simulink model "flightControlSystem"  (R2021a)
settings: Solver=ode3  StartTime=0  StopTime=TFinal  FixedStep=Ts  RelTol=1e-3  EnableMultiTasking=on
undefined symbols (not defined in the file): codertarget, Estimator, Ts
libraries: simulink x6
settings Model: ExtModeTrigDuration=80  Creator=The MathWorks, Inc.  LastModifiedBy=s2130866
settings SolverCC: AlgebraicLoopSolver=TrustRegion
settings DataIOCC: LimitDataPoints=on  SaveFormat=StructureWithTime  ReturnWorkspaceOutputs=off
settings OptimizationCC: BlockReduction=off  EnhancedBackFolding=on  PassReuseOutputArgsAs=Individual arguments  ZeroExternalMemoryAtStartup=off  ZeroInternalMemoryAtStartup=off  MaxStackSize=64  OptimizeBlockOrder=speed  DifferentSizesBufferReuse=on  OptimizationCustomize=off  EfficientTunableParamExpr=on
settings DebuggingCC: AlgebraicLoopMsg=none  IntegerOverflowMsg=none  ParameterPrecisionLossMsg=none  ParameterTunabilityLossMsg=error  UnconnectedInputMsg=none  UnconnectedOutputMsg=none  UnconnectedLineMsg=none  BusObjectLabelMismatch=error  SFUnexpectedBacktrackingDiag=warning  SFNoUnconditionalDefaultTransitionDiag=warning  SFExecutionAtInitializationDiag=none  SFMachineParentedDataDiag=warning  IntegerSaturationMsg=none  ArithmeticOperatorsInVariantConditions=warning
settings HardwareCC: ProdBitPerPointer=32  ProdBitPerSizeT=32  ProdBitPerPtrDiffT=32  ProdLargestAtomicInteger=Long  ProdWordSize=32  ProdHWDeviceType=ARM Compatible->ARM 9
settings ModelReferenceCC: ModelReferenceNumInstancesAllowed=Single  PropagateSignalLabelsOutOfModel=off
settings SFSimCC: SimUseLocalCustomCode=off  MATLABDynamicMemAlloc=off  CustomCodeUndefinedFunction=UseInterfaceOnly
settings RTWCC: SystemTargetFile=ert.tlc  HardwareBoard=PARROT Mambo  TemplateMakefile=ert_default_tmf  GenerateReport=on  RTWUseLocalCustomCode=off  Toolchain=Sourcery G++ Lite GNU Toolchain for Drones  LaunchReport=on
settings CodeAppCC: ForceParamTrailComments=on  IgnoreCustomStorageClasses=off  MaxIdLength=63  OperatorAnnotations=on  SimulinkDataObjDesc=on  SFDataObjDesc=on  InsertBlockDesc=on
settings ERTTargetCC: MatFileLogging=on
settings ConfigComp: CovMetricSettings=dw  CovSaveCumulativeToWorkspaceVar=on  CovSaveSingleToWorkspaceVar=on  CovExternalEMLEnable=off  CovSFcnEnable=off

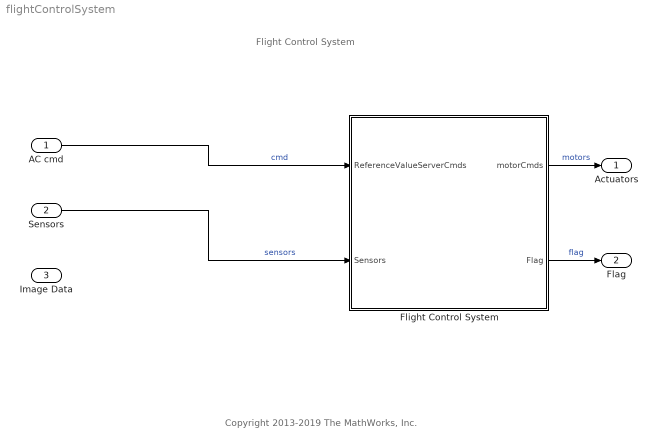
== system flightControlSystem ==
  note: Copyright 2013-2019 The MathWorks, Inc.
  note: Flight Control System
  AC cmd : Inport  OutDataTypeStr=Bus: CommandBus  BusOutputAsStruct=on
  Sensors : Inport  Port=2  OutDataTypeStr=Bus: SensorsBus  BusOutputAsStruct=on
  Image Data : Inport  Tag=IP_IN  InitFcn=codertarget.parrot.internal.inportCallback(gcb);  Port=3  OutDataTypeStr=uint8  PortDimensions=[4 9600]  BusOutputAsStruct=on
  Flight Control System : Subsystem  TreatAsAtomicUnit=on  SystemSampleTime=Ts
  Actuators : Outport  OutDataTypeStr=single  PortDimensions=4  VectorParamsAs1DForOutWhenUnconnected=off
  Flag : Outport  Port=2  OutDataTypeStr=uint8  PortDimensions=1  VectorParamsAs1DForOutWhenUnconnected=off
  wires:
  AC cmd/1 -> Flight Control System/1(ReferenceValueServerCmds)  "cmd"
  Flight Control System/1(motorCmds) -> Actuators/1  "motors"
  Sensors/1 -> Flight Control System/2(Sensors)  "sensors"
  Flight Control System/2(Flag) -> Flag/1  "flag"

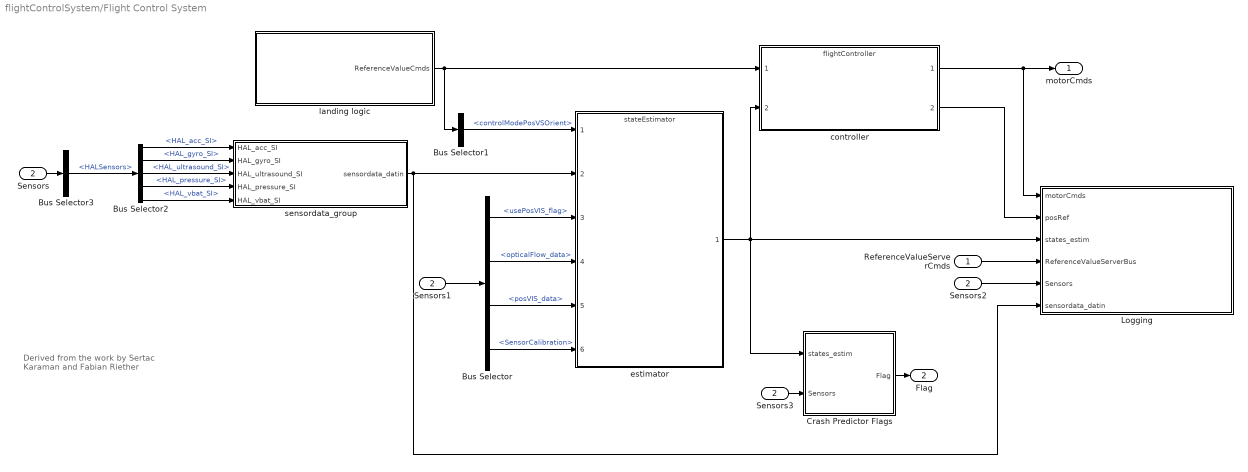
== system flightControlSystem/Flight Control System ==
  note: Derived from the work by Sertac
      | Karaman and Fabian Riether
  ReferenceValueServerCmds : Inport  OutDataTypeStr=Bus: CommandBus
  Sensors : Inport  Port=2  OutDataTypeStr=Bus: SensorsBus  BusOutputAsStruct=on
  Bus Selector : BusSelector  OutputSignals=VisionSensors.usePosVIS_flag,VisionSensors.opticalFlow_data,VisionSensors.posVIS_data,SensorCalibration
  Bus Selector1 : BusSelector  OutputSignals=controlModePosVSOrient
  Bus Selector2 : BusSelector  OutputSignals=HAL_acc_SI,HAL_gyro_SI,HAL_ultrasound_SI,HAL_pressure_SI,HAL_vbat_SI
  Bus Selector3 : BusSelector  OutputSignals=HALSensors
  Crash Predictor Flags : Subsystem
  Logging : Subsystem  TreatAsAtomicUnit=on
      settings: RTWFcnNameOpts=Use subsystem name
  Sensors1 : InportShadow  Port=2  OutDataTypeStr=Bus: SensorsBus  BusOutputAsStruct=on
  Sensors2 : InportShadow  Port=2  OutDataTypeStr=Bus: SensorsBus  BusOutputAsStruct=on
  Sensors3 : InportShadow  Port=2  OutDataTypeStr=Bus: SensorsBus  BusOutputAsStruct=on
  controller : ModelReference  ModelNameDialog=flightController.slx  SimulationMode=Normal  ModelReferenceVersion=4.1
  estimator : ModelReference  ModelNameDialog=stateEstimator.slx  SimulationMode=Normal  ModelReferenceVersion=4.1
  landing logic : Subsystem
  sensordata_group : Subsystem
  motorCmds : Outport  VectorParamsAs1DForOutWhenUnconnected=off
  Flag : Outport  Port=2  VectorParamsAs1DForOutWhenUnconnected=off
  wires:
  Bus Selector2/1 -> sensordata_group/1(HAL_acc_SI)  "<HAL_acc_SI>"
  Bus Selector2/2 -> sensordata_group/2(HAL_gyro_SI)  "<HAL_gyro_SI>"
  Bus Selector2/4 -> sensordata_group/4(HAL_pressure_SI)  "<HAL_pressure_SI>"
  Bus Selector2/3 -> sensordata_group/3(HAL_ultrasound_SI)  "<HAL_ultrasound_SI>"
  estimator/1 -> Crash Predictor Flags/1(states_estim), Logging/3(states_estim), controller/2
  Sensors2/1 -> Logging/5(Sensors)
  controller/2 -> Logging/2(posRef)
  ReferenceValueServerCmds/1 -> Logging/4(ReferenceValueServerBus)
  controller/1 -> Logging/1(motorCmds), motorCmds/1
  sensordata_group/1(sensordata_datin) -> Logging/6(sensordata_datin), estimator/2
  Bus Selector2/5 -> sensordata_group/5(HAL_vbat_SI)  "<HAL_vbat_SI>"
  Crash Predictor Flags/1(Flag) -> Flag/1
  Sensors/1 -> Bus Selector3/1
  Bus Selector3/1 -> Bus Selector2/1  "<HALSensors>"
  Sensors1/1 -> Bus Selector/1
  Bus Selector/1 -> estimator/3  "<usePosVIS_flag>"
  Bus Selector/2 -> estimator/4  "<opticalFlow_data>"
  Bus Selector/3 -> estimator/5  "<posVIS_data>"
  Bus Selector/4 -> estimator/6  "<SensorCalibration>"
  Bus Selector1/1 -> estimator/1  "<controlModePosVSOrient>"
  landing logic/1(ReferenceValueCmds) -> Bus Selector1/1, controller/1
  Sensors3/1 -> Crash Predictor Flags/2(Sensors)

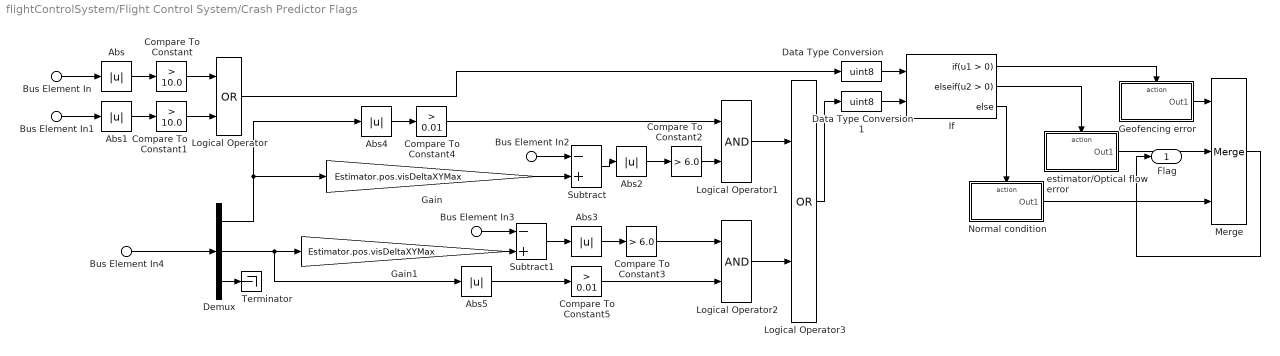
== system flightControlSystem/Flight Control System/Crash Predictor Flags ==
  Bus Element In : Inport  PortName=states_estim  Element=X
  Bus Element In1 : Inport  PortName=states_estim  Element=Y
  Bus Element In2 : Inport  PortName=states_estim  Element=dx
  Bus Element In3 : Inport  PortName=states_estim  Element=dy
  Bus Element In4 : Inport  Port=2  PortName=Sensors  Element=VisionSensors.opticalFlow_data
  Abs{,1..5} (6 alike) : Abs
  Compare To Constant : simulink/Logic and Bit Operations/Compare To Constant  relop=>  const=10.0  OutDataTypeStr=boolean
  Compare To Constant1 : simulink/Logic and Bit Operations/Compare To Constant  relop=>  const=10.0  OutDataTypeStr=boolean
  Compare To Constant2 : simulink/Logic and Bit Operations/Compare To Constant  relop=>  const=6.0  OutDataTypeStr=boolean
  Compare To Constant3 : simulink/Logic and Bit Operations/Compare To Constant  relop=>  const=6.0  OutDataTypeStr=boolean
  Compare To Constant4 : simulink/Logic and Bit Operations/Compare To Constant  relop=>  const=0.01  OutDataTypeStr=boolean
  Compare To Constant5 : simulink/Logic and Bit Operations/Compare To Constant  relop=>  const=0.01  OutDataTypeStr=boolean
  Data Type Conversion : DataTypeConversion  OutDataTypeStr=uint8  RndMeth=Nearest
  Data Type Conversion1 : DataTypeConversion  OutDataTypeStr=uint8  RndMeth=Nearest
  Demux : Demux  Outputs=3
  Gain : Gain  Gain=Estimator.pos.visDeltaXYMax
  Gain1 : Gain  Gain=Estimator.pos.visDeltaXYMax
  Geofencing error : Subsystem  TreatAsAtomicUnit=on
  If : If  NumInputs=2  ElseIfExpressions=u2 > 0
  Logical Operator : Logic  Operator=OR  AllPortsSameDT=off
  Logical Operator1 : Logic  AllPortsSameDT=off  OutDataTypeStr=boolean
  Logical Operator2 : Logic  AllPortsSameDT=off  OutDataTypeStr=boolean
  Logical Operator3 : Logic  Operator=OR  AllPortsSameDT=off
  Merge : Merge  Inputs=3  InitialOutput=0
  Normal condition : Subsystem  TreatAsAtomicUnit=on
  Subtract : Sum  Inputs=-+
  Subtract1 : Sum  Inputs=-+
  Terminator : Terminator
  estimator/Optical flow error : Subsystem  TreatAsAtomicUnit=on
  Flag : Outport  VectorParamsAs1DForOutWhenUnconnected=off
  wires:
  Bus Element In/1 -> Abs/1
  Bus Element In1/1 -> Abs1/1
  Compare To Constant/1 -> Logical Operator/1
  Compare To Constant1/1 -> Logical Operator/2
  Abs/1 -> Compare To Constant/1
  Abs1/1 -> Compare To Constant1/1
  Logical Operator/1 -> Data Type Conversion/1
  Demux/1 -> Abs4/1, Gain/1
  Demux/2 -> Gain1/1, Abs5/1
  Bus Element In2/1 -> Subtract/1
  Subtract/1 -> Abs2/1
  Subtract1/1 -> Abs3/1
  Abs2/1 -> Compare To Constant2/1
  Abs3/1 -> Compare To Constant3/1
  Compare To Constant5/1 -> Logical Operator2/2
  Abs4/1 -> Compare To Constant4/1
  Abs5/1 -> Compare To Constant5/1
  Compare To Constant3/1 -> Logical Operator2/1
  Logical Operator1/1 -> Logical Operator3/1
  Logical Operator2/1 -> Logical Operator3/2
  Logical Operator3/1 -> Data Type Conversion1/1
  Demux/3 -> Terminator/1
  Gain/1 -> Subtract/2
  Bus Element In3/1 -> Subtract1/1
  Gain1/1 -> Subtract1/2
  Compare To Constant4/1 -> Logical Operator1/1
  Compare To Constant2/1 -> Logical Operator1/2
  Merge/1 -> Flag/1
  If/1 -> Geofencing error/Action
  If/2 -> estimator/Optical flow error/Action
  If/3 -> Normal condition/Action
  Geofencing error/1(Out1) -> Merge/1
  estimator/Optical flow error/1(Out1) -> Merge/2
  Normal condition/1(Out1) -> Merge/3
  Data Type Conversion/1 -> If/1
  Data Type Conversion1/1 -> If/2
  Bus Element In4/1 -> Demux/1

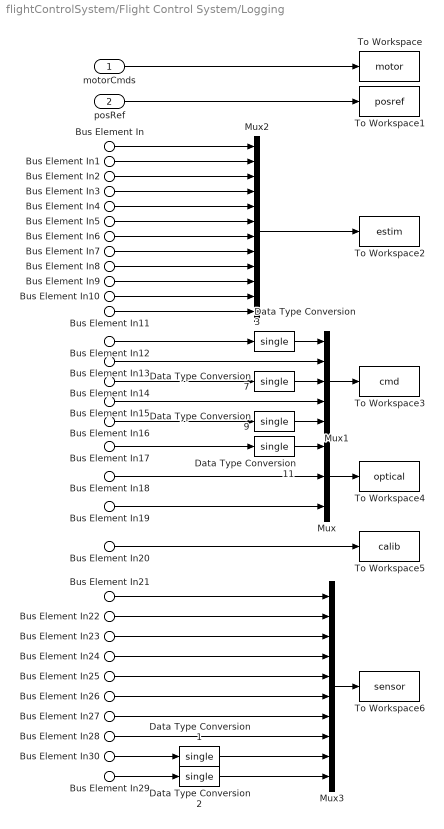
== system flightControlSystem/Flight Control System/Logging ==
  motorCmds : Inport
  posRef : Inport  Port=2
  Bus Element In : Inport  Port=3  PortName=states_estim  Element=X
  Bus Element In1 : Inport  Port=3  PortName=states_estim  Element=Y
  Bus Element In2 : Inport  Port=3  PortName=states_estim  Element=Z
  Bus Element In3 : Inport  Port=3  PortName=states_estim  Element=yaw
  Bus Element In6 : Inport  Port=3  PortName=states_estim  Element=dx
  Bus Element In5 : Inport  Port=3  PortName=states_estim  Element=roll
  Bus Element In4 : Inport  Port=3  PortName=states_estim  Element=pitch
  Bus Element In7 : Inport  Port=3  PortName=states_estim  Element=dy
  Bus Element In8 : Inport  Port=3  PortName=states_estim  Element=dz
  Bus Element In9 : Inport  Port=3  PortName=states_estim  Element=p
  Bus Element In10 : Inport  Port=3  PortName=states_estim  Element=q
  Bus Element In11 : Inport  Port=3  PortName=states_estim  Element=r
  Bus Element In12 : Inport  Port=4  PortName=ReferenceValueServerBus  Element=controlModePosVSOrient
  Bus Element In13 : Inport  Port=4  PortName=ReferenceValueServerBus  Element=pos_ref
  Bus Element In14 : Inport  Port=4  PortName=ReferenceValueServerBus  Element=takeoff_flag
  Bus Element In15 : Inport  Port=4  PortName=ReferenceValueServerBus  Element=orient_ref
  Bus Element In16 : Inport  Port=4  PortName=ReferenceValueServerBus  Element=live_time_ticks
  Bus Element In17 : Inport  Port=5  PortName=Sensors  Element=VisionSensors.usePosVIS_flag
  Bus Element In18 : Inport  Port=5  PortName=Sensors  Element=VisionSensors.opticalFlow_data
  Bus Element In19 : Inport  Port=5  PortName=Sensors  Element=VisionSensors.posVIS_data
  Bus Element In20 : Inport  Port=5  PortName=Sensors  Element=SensorCalibration
  Bus Element In21 : Inport  Port=6  PortName=sensordata_datin  Element=ddx
  Bus Element In22 : Inport  Port=6  PortName=sensordata_datin  Element=ddy
  Bus Element In23 : Inport  Port=6  PortName=sensordata_datin  Element=ddz
  Bus Element In24 : Inport  Port=6  PortName=sensordata_datin  Element=p
  Bus Element In25 : Inport  Port=6  PortName=sensordata_datin  Element=q
  Bus Element In26 : Inport  Port=6  PortName=sensordata_datin  Element=r
  Bus Element In27 : Inport  Port=6  PortName=sensordata_datin  Element=altitude_sonar
  Bus Element In28 : Inport  Port=6  PortName=sensordata_datin  Element=prs
  Bus Element In29 : Inport  Port=6  PortName=sensordata_datin  Element=vbat_percentage
  Bus Element In30 : Inport  Port=6  PortName=sensordata_datin  Element=vbat_V
  Data Type Conversion{1..3,7,9,11} (6 alike) : DataTypeConversion  OutDataTypeStr=single
  Mux : Mux  Inputs=3
  Mux1 : Mux  Inputs=5
  Mux2 : Mux  Inputs=12
  Mux3 : Mux  Inputs=10
  To Workspace : ToWorkspace  VariableName=motor  SaveFormat=Structure With Time  SampleTime=-1
  To Workspace1 : ToWorkspace  VariableName=posref  SaveFormat=Structure With Time  SampleTime=-1
  To Workspace2 : ToWorkspace  VariableName=estim  SaveFormat=Structure With Time  SampleTime=-1
  To Workspace3 : ToWorkspace  VariableName=cmd  SaveFormat=Structure With Time  SampleTime=-1
  To Workspace4 : ToWorkspace  VariableName=optical  SaveFormat=Structure With Time  SampleTime=-1
  To Workspace5 : ToWorkspace  VariableName=calib  SaveFormat=Structure With Time  SampleTime=-1
      settings: Decimation=100
  To Workspace6 : ToWorkspace  VariableName=sensor  SaveFormat=Structure With Time  SampleTime=-1
  wires:
  Bus Element In12/1 -> Data Type Conversion3/1
  Bus Element In14/1 -> Data Type Conversion7/1
  Bus Element In16/1 -> Data Type Conversion9/1
  Bus Element In17/1 -> Data Type Conversion11/1
  Bus Element In20/1 -> To Workspace5/1
  Mux/1 -> To Workspace4/1
  Mux2/1 -> To Workspace2/1
  motorCmds/1 -> To Workspace/1
  Mux1/1 -> To Workspace3/1
  Bus Element In3/1 -> Mux2/4
  Bus Element In5/1 -> Mux2/6
  Bus Element In4/1 -> Mux2/5
  Bus Element In8/1 -> Mux2/9
  Bus Element In6/1 -> Mux2/7
  Bus Element In7/1 -> Mux2/8
  Bus Element In9/1 -> Mux2/10
  Bus Element In11/1 -> Mux2/12
  Bus Element In1/1 -> Mux2/2
  Bus Element In10/1 -> Mux2/11
  Bus Element In2/1 -> Mux2/3
  Bus Element In/1 -> Mux2/1
  Data Type Conversion3/1 -> Mux1/1
  Bus Element In13/1 -> Mux1/2
  Data Type Conversion7/1 -> Mux1/3
  Bus Element In15/1 -> Mux1/4
  Data Type Conversion9/1 -> Mux1/5
  Bus Element In19/1 -> Mux/3
  Bus Element In18/1 -> Mux/2
  Data Type Conversion11/1 -> Mux/1
  posRef/1 -> To Workspace1/1
  Bus Element In21/1 -> Mux3/1
  Bus Element In22/1 -> Mux3/2
  Bus Element In23/1 -> Mux3/3
  Bus Element In24/1 -> Mux3/4
  Bus Element In25/1 -> Mux3/5
  Bus Element In26/1 -> Mux3/6
  Bus Element In27/1 -> Mux3/7
  Bus Element In28/1 -> Mux3/8
  Bus Element In30/1 -> Data Type Conversion1/1
  Bus Element In29/1 -> Data Type Conversion2/1
  Mux3/1 -> To Workspace6/1
  Data Type Conversion1/1 -> Mux3/9
  Data Type Conversion2/1 -> Mux3/10

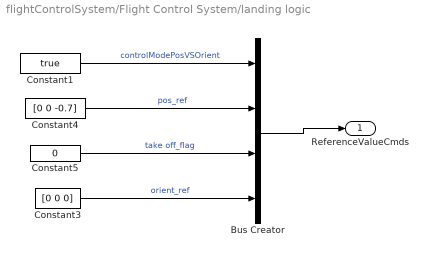
== system flightControlSystem/Flight Control System/landing logic ==
  Bus Creator : BusCreator  Inputs=4  OutDataTypeStr=Bus: CommandBus
  Constant1 : Constant  Value=true  OutDataTypeStr=boolean
  Constant3 : Constant  Value=[0 0 0]  OutDataTypeStr=single
  Constant4 : Constant  Value=[0 0 -0.7]  OutDataTypeStr=single
  Constant5 : Constant  Value=0  OutDataTypeStr=boolean
  ReferenceValueCmds : Outport  OutDataTypeStr=Bus: CommandBus  VectorParamsAs1DForOutWhenUnconnected=off
  wires:
  Constant4/1 -> Bus Creator/2  "pos_ref"
  Constant1/1 -> Bus Creator/1  "controlModePosVSOrient"
  Constant5/1 -> Bus Creator/3  "take off_flag"
  Constant3/1 -> Bus Creator/4  "orient_ref"
  Bus Creator/1 -> ReferenceValueCmds/1

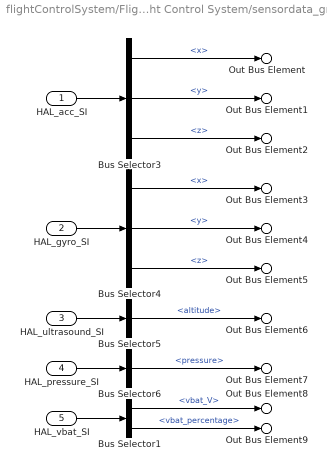
== system flightControlSystem/Flight Control System/sensordata_group ==
  HAL_acc_SI : Inport  OutDataTypeStr=Bus: HAL_acc_SI_t
  HAL_gyro_SI : Inport  Port=2  OutDataTypeStr=Bus: HAL_gyro_SI_t
  HAL_ultrasound_SI : Inport  Port=3  OutDataTypeStr=Bus: HAL_ultrasound_SI_t
  HAL_pressure_SI : Inport  Port=4  OutDataTypeStr=Bus: HAL_pressure_SI_t
  HAL_vbat_SI : Inport  Port=5  OutDataTypeStr=Bus: HAL_vbat_SI_t
  Bus Selector1 : BusSelector  OutputSignals=vbat_V,vbat_percentage
  Bus Selector3 : BusSelector  OutputSignals=x,y,z
  Bus Selector4 : BusSelector  OutputSignals=x,y,z
  Bus Selector5 : BusSelector  OutputSignals=altitude
  Bus Selector6 : BusSelector  OutputSignals=pressure
  Out Bus Element : Outport  VectorParamsAs1DForOutWhenUnconnected=off  PortName=sensordata_datin  Element=ddx
  Out Bus Element1 : Outport  VectorParamsAs1DForOutWhenUnconnected=off  PortName=sensordata_datin  Element=ddy
  Out Bus Element2 : Outport  VectorParamsAs1DForOutWhenUnconnected=off  PortName=sensordata_datin  Element=ddz
  Out Bus Element3 : Outport  VectorParamsAs1DForOutWhenUnconnected=off  PortName=sensordata_datin  Element=p
  Out Bus Element4 : Outport  VectorParamsAs1DForOutWhenUnconnected=off  PortName=sensordata_datin  Element=q
  Out Bus Element5 : Outport  VectorParamsAs1DForOutWhenUnconnected=off  PortName=sensordata_datin  Element=r
  Out Bus Element6 : Outport  VectorParamsAs1DForOutWhenUnconnected=off  PortName=sensordata_datin  Element=altitude_sonar
  Out Bus Element7 : Outport  VectorParamsAs1DForOutWhenUnconnected=off  PortName=sensordata_datin  Element=prs
  Out Bus Element8 : Outport  VectorParamsAs1DForOutWhenUnconnected=off  PortName=sensordata_datin  Element=vbat_V
  Out Bus Element9 : Outport  VectorParamsAs1DForOutWhenUnconnected=off  PortName=sensordata_datin  Element=vbat_percentage
  wires:
  HAL_gyro_SI/1 -> Bus Selector4/1
  HAL_acc_SI/1 -> Bus Selector3/1
  HAL_pressure_SI/1 -> Bus Selector6/1
  HAL_ultrasound_SI/1 -> Bus Selector5/1
  Bus Selector4/1 -> Out Bus Element3/1  "<x>"
  Bus Selector3/3 -> Out Bus Element2/1  "<z>"
  Bus Selector4/3 -> Out Bus Element5/1  "<z>"
  Bus Selector5/1 -> Out Bus Element6/1  "<altitude>"
  Bus Selector6/1 -> Out Bus Element7/1  "<pressure>"
  Bus Selector4/2 -> Out Bus Element4/1  "<y>"
  Bus Selector3/1 -> Out Bus Element/1  "<x>"
  Bus Selector3/2 -> Out Bus Element1/1  "<y>"
  Bus Selector1/1 -> Out Bus Element8/1  "<vbat_V>"
  HAL_vbat_SI/1 -> Bus Selector1/1
  Bus Selector1/2 -> Out Bus Element9/1  "<vbat_percentage>"

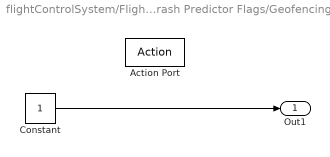
== system flightControlSystem/Flight Control System/Crash Predictor Flags/Geofencing error ==
  Action Port : ActionPort  ActionPortLabel=if(u1 > 0)
  Constant : Constant  OutDataTypeStr=uint8
  Out1 : Outport  VectorParamsAs1DForOutWhenUnconnected=off
  wires:
  Constant/1 -> Out1/1

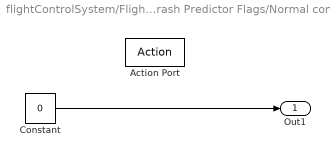
== system flightControlSystem/Flight Control System/Crash Predictor Flags/Normal condition ==
  Action Port : ActionPort  ActionPortLabel=else
  Constant : Constant  Value=0  OutDataTypeStr=uint8
  Out1 : Outport  VectorParamsAs1DForOutWhenUnconnected=off
  wires:
  Constant/1 -> Out1/1

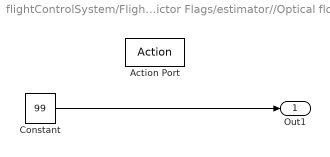
== system flightControlSystem/Flight Control System/Crash Predictor Flags/estimator//Optical flow error ==
  Action Port : ActionPort  ActionPortLabel=elseif(u2 > 0)
  Constant : Constant  Value=99  OutDataTypeStr=uint8
  Out1 : Outport  VectorParamsAs1DForOutWhenUnconnected=off
  wires:
  Constant/1 -> Out1/1
